simulink subsystem "BUF_MIN_MAX_AVG_fixed"  (R2024a)
settings: Solver=VariableStepAuto  StartTime=0.0  StopTime=10.0  RelTol=1e-3
values from neighbouring files (symbols this model uses):
  BUFFER_LEN = 2048    [workspace.mat]
  SAMPLING_FREQ = 12800    [workspace.mat]
libraries: dspsigops x3, hdlsllib x1, simulink_extras x1
settings Model: Creator=Jan Rosa  LastModifiedBy=Jan Rosa

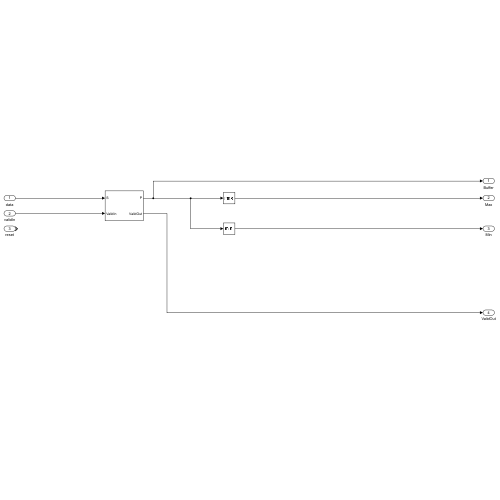
[thumbnail: Simulink's stored preview of the top-level diagram]
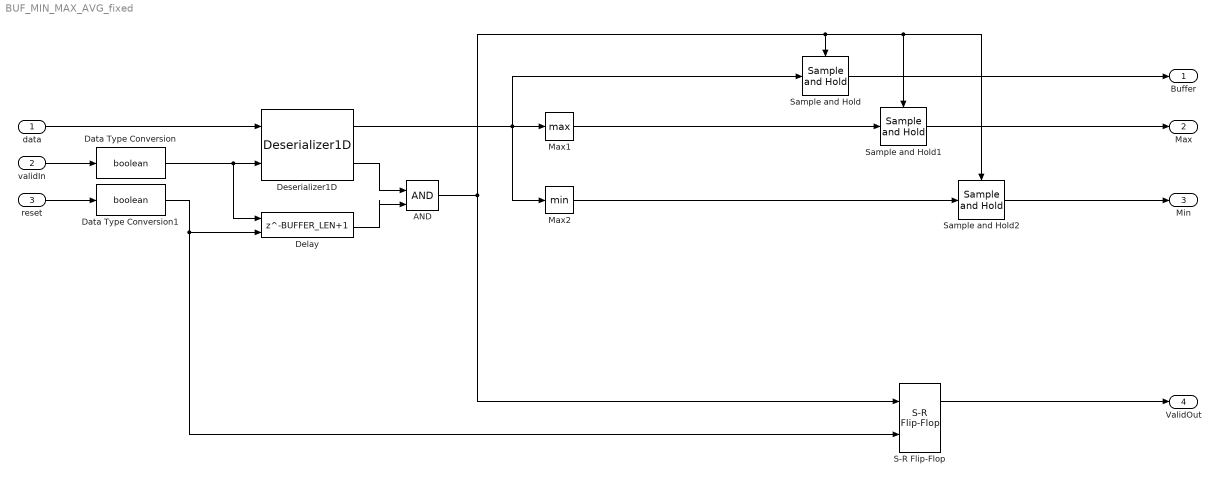
== system BUF_MIN_MAX_AVG_fixed ==
  data : Inport  OutDataTypeStr=fixdt(1,16,14)
  validIn : Inport  Port=2  OutDataTypeStr=fixdt(1,16,14)
  reset : Inport  Port=3  OutDataTypeStr=fixdt(1,16,14)
  AND : Logic  IconShape=distinctive  AllPortsSameDT=off  OutDataTypeStr=boolean
  Data Type Conversion : DataTypeConversion  OutDataTypeStr=boolean  SaturateOnIntegerOverflow=off  RndMeth=Floor
  Data Type Conversion1 : DataTypeConversion  OutDataTypeStr=boolean  SaturateOnIntegerOverflow=off  RndMeth=Floor
  Delay : Delay  DelayLength=BUFFER_LEN+1  ExternalReset=Rising
      settings: InputPortMap=u0,r5
  Deserializer1D : hdlsllib/HDL Operations/Deserializer1D  Ratio=BUFFER_LEN  IdleCycles=0  InitialCondition=0  startIn=off  validIn=on  validOut=on  inputDataDimensions=1  inputSampleTime=1/SAMPLING_FREQ  inputSignalType=auto
  Max1 : MinMax  Function=max  OutDataTypeStr=fixdt(0,16,16)
  Max2 : MinMax  OutDataTypeStr=fixdt(1,16,15)
  S-R Flip-Flop : simulink_extras/Flip Flops/S-R Flip-Flop  initial_condition=0
  Sample and Hold : dspsigops/Sample and Hold  trig=Rising edge  initCond=0  latchinput=off
  Sample and Hold1 : dspsigops/Sample and Hold  trig=Rising edge  initCond=0  latchinput=off
  Sample and Hold2 : dspsigops/Sample and Hold  trig=Rising edge  initCond=0  latchinput=off
  Buffer : Outport
  Max : Outport  Port=2
  Min : Outport  Port=3
  ValidOut : Outport  Port=4
  wires:
  Deserializer1D/1 -> Max1/1, Max2/1, Sample and Hold/1
  Deserializer1D/2 -> AND/1
  validIn/1 -> Data Type Conversion/1
  data/1 -> Deserializer1D/1
  Data Type Conversion/1 -> Deserializer1D/2, Delay/1
  Sample and Hold/1 -> Buffer/1
  Max2/1 -> Sample and Hold2/1
  Max1/1 -> Sample and Hold1/1
  Sample and Hold1/1 -> Max/1
  Sample and Hold2/1 -> Min/1
  AND/1 -> Sample and Hold/Trigger, Sample and Hold2/Trigger, Sample and Hold1/Trigger, S-R Flip-Flop/1
  reset/1 -> Data Type Conversion1/1
  S-R Flip-Flop/1 -> ValidOut/1
  Delay/1 -> AND/2
  Data Type Conversion1/1 -> S-R Flip-Flop/2, Delay/2
